simulink model "BLDC_180deg_hall_misalign"  (R2024a)
settings: Solver=ode15s  StartTime=0.0  StopTime=10  RelTol=1e-3
undefined symbols (not defined in the file or in its folder): HallError1, HallError2, HallError3, WrappedHallError1
libraries: simulink x10, dspswit3 x2, slpidlib x1
settings Model: Creator=matthewhasman  LastModifiedBy=matthewhasman

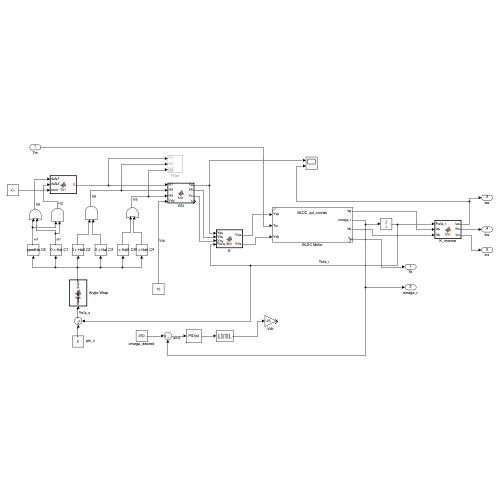
[thumbnail: Simulink's stored preview of the top-level diagram]
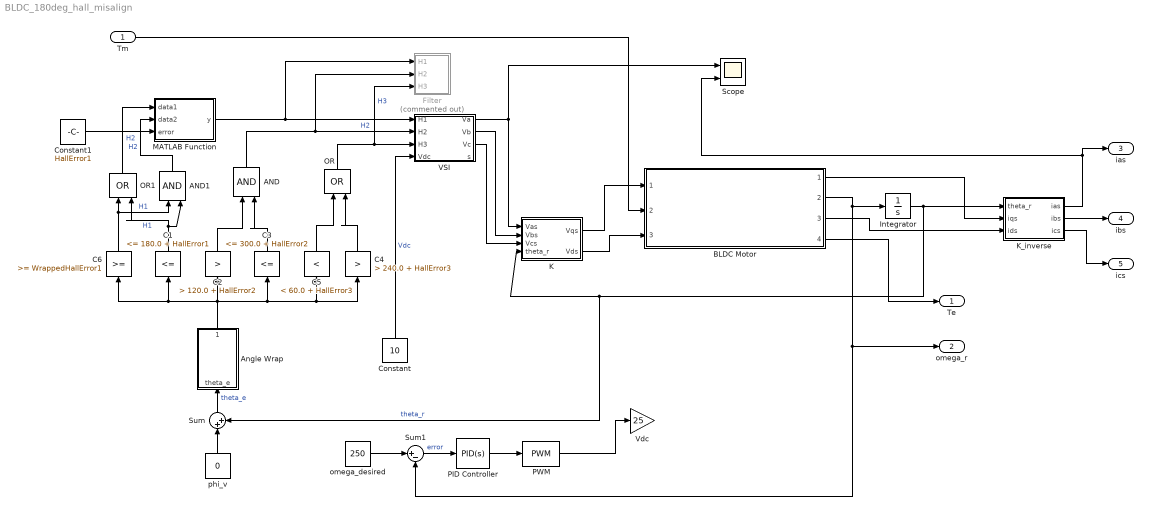
== system BLDC_180deg_hall_misalign ==
  Tm : Inport
  AND : Logic  IconShape=distinctive  AllPortsSameDT=off  OutDataTypeStr=boolean
  AND1 : Logic  IconShape=distinctive  AllPortsSameDT=off  OutDataTypeStr=boolean
  Angle Wrap : MATLAB Function  TreatAsAtomicUnit=on
  BLDC Motor : Subsystem  ReferencedSubsystem=BLDC_qd_coords
  C1 : simulink/Logic and Bit Operations/Compare To Constant  relop=<=  const=180.0 + HallError1  OutDataTypeStr=boolean
  C2 : simulink/Logic and Bit Operations/Compare To Constant  relop=>  const=120.0 + HallError2  OutDataTypeStr=boolean
  C3 : simulink/Logic and Bit Operations/Compare To Constant  relop=<=  const=300.0 + HallError2  OutDataTypeStr=boolean
  C4 : simulink/Logic and Bit Operations/Compare To Constant  relop=>  const=240.0 + HallError3  OutDataTypeStr=boolean
  C5 : simulink/Logic and Bit Operations/Compare To Constant  relop=<  const=60.0 + HallError3  OutDataTypeStr=boolean
  C6 : simulink/Logic and Bit Operations/Compare To Constant  relop=>=  const=WrappedHallError1  OutDataTypeStr=boolean
  Constant : Constant  Value=10
  Constant1 : Constant  Value=HallError1
  Filter : Subsystem  Commented=on
  Integrator : Integrator
  K : MATLAB Function  TreatAsAtomicUnit=on
  K_inverse : MATLAB Function  TreatAsAtomicUnit=on
  MATLAB Function : MATLAB Function  TreatAsAtomicUnit=on
  OR : Logic  Operator=OR  IconShape=distinctive  AllPortsSameDT=off  OutDataTypeStr=boolean
  OR1 : Logic  Operator=OR  IconShape=distinctive  AllPortsSameDT=off  OutDataTypeStr=boolean
  PID Controller : slpidlib/PID Controller  Controller=PID  Form=Parallel  TimeDomain=Continuous-time  UseExternalTs=off  SampleTime=-1  IntegratorMethod=Forward Euler  FilterMethod=Forward Euler  ControllerParametersSource=internal  P=8  I=5  UseKiTs=off  D=1  UseExternalDerivativeSource=off  N=100  UseFilter=on  TunerSelectOption=Transfer Function Based (PID Tuner App)  InitialConditionSource=internal  InitialConditionForIntegrator=0  InitialConditionForFilter=0  DifferentiatorICPrevScaledInput=0  ExternalReset=none  TrackingMode=off  Kt=1  LimitOutput=off  SatLimitsSource=internal  UpperSaturationLimit=inf  LowerSaturationLimit=-inf  LinearizeAsGain=on  AntiWindupMode=none  Kb=1  LimitIntegrator=off  UpperIntegratorSaturationLimit=inf  LowerIntegratorSaturationLimit=-inf  POutMin=[]  POutMax=[]  IOutMin=[]  IOutMax=[]  DOutMin=[]  DOutMax=[]  NOutMin=[]  NOutMax=[]  SumOutMin=[]  SumOutMax=[]  SaturationOutMin=[]  SaturationOutMax=[]  PParamMin=[]  PParamMax=[]  IParamMin=[]  IParamMax=[]  DParamMin=[]  DParamMax=[]  NParamMin=[]  NParamMax=[]  KbParamMin=[]  KbParamMax=[]  KtParamMin=[]  KtParamMax=[]  KbOutMin=[]  KbOutMax=[]  KtOutMin=[]  KtOutMax=[]  IntegratorOutMin=[]  IntegratorOutMax=[]  FilterOutMin=[]  FilterOutMax=[]  SumI1OutMin=[]  SumI1OutMax=[]  SumI2OutMin=[]  SumI2OutMax=[]  SumI3OutMin=[]  SumI3OutMax=[]  SumI4OutMin=[]  SumI4OutMax=[]  SumDOutMin=[]  SumDOutMax=[]  DifferentiatorOutMin=[]  DifferentiatorOutMax=[]  FilterDiffOutCoefMin=[]  FilterDiffOutCoefMax=[]  ReciprocalOutMin=[]  ReciprocalOutMax=[]  SumDenOutMin=[]  SumDenOutMax=[]  SumNumOutMin=[]  SumNumOutMax=[]  DivideOutMin=[]  DivideOutMax=[]  UdiffTsProdOutMin=[]  UdiffTsProdOutMax=[]  NTsProdOutMin=[]  NTsProdOutMax=[]  UintegralTsProdOutMin=[]  UintegralTsProdOutMax=[]  UngainTsProdOutMin=[]  UngainTsProdOutMax=[]  ClampingZeroOutDataTypeStr=Inherit: Inherit via back propagation  ClampingZeroOutMin=[]  ClampingZeroOutMax=[]  FilterDenConstantOutDataTypeStr=Inherit: Inherit via back propagation  FilterDenConstantOutMin=[]  FilterDenConstantOutMax=[]  PCopyOutDataTypeStr=Inherit: Inherit via back propagation  PCopyOutMin=[]  PCopyOutMax=[]  NCopyOutDataTypeStr=Inherit: Inherit via back propagation  NCopyOutMin=[]  NCopyOutMax=[]  IntegratorContinuousStateAttributes=''  IntegratorStateMustResolveToSignalObject=off  IntegratorRTWStateStorageClass=Auto  FilterContinuousStateAttributes=''  FilterStateMustResolveToSignalObject=off  FilterRTWStateStorageClass=Auto  ParallelPVariant=InternalParameters  IdealPVariant=Disabled  IVariant=InternalParameters  DVariant=InternalParameters  IntegratorVariant=Continuous  SatVariant=Disabled  AWVariant=Passthrough  PCopyVariant=Disabled  TRVariant=Disabled  FdbkBlocksVariant=Forward  IdealPFdbkVariant=Disabled  SatFdbkVariant=Disabled  DerivativeFilterVariant=ContFilter  NVariant=InternalParameters  NCopyVariant=Disabled  FilterICVariant=InternalICsFilter  IntegratorICVariant=InternalICs  ExternalResetVariant=Disabled  TRSumVariant=Passthrough  SumFdbkVariant=Disabled  SumVariant=Sum_PID  TsampFilterVariant=InternalTs  TsampNgainVariant=Passthrough  TsampIntegralVariant=Disabled_SignalSpec  ExternalSaturationOutDataTypeStr=Inherit: Same as second input  DerivativeSourceVariant=ErrorSignal
  PWM : simulink/Discontinuities/PWM  DisableCoverage=on  Period=0.0001  InitialDelay=0  DisallowZeroDutyCycle=off  RunAtFixedTimeIntervals=off  SampleTime=0.1
  Scope : Scope  NumInputPorts=2
  Sum : Sum  Inputs=|++
  Sum1 : Sum  Inputs=|+-
  VSI : MATLAB Function  TreatAsAtomicUnit=on
  Vdc : Gain  Gain=25
  omega_desired : Constant  Value=250
  phi_v : Constant  Value=0
  Te : Outport
  omega_r : Outport  Port=2
  ias : Outport  Port=3
  ibs : Outport  Port=4
  ics : Outport  Port=5
  wires:
  Integrator/1 -> K_inverse/1(theta_r), K/4(theta_r), Sum/2  "theta_r"
  BLDC Motor/1 -> K_inverse/2(iqs)
  BLDC Motor/3 -> K_inverse/3(ids)
  K/1(Vqs) -> BLDC Motor/1
  Tm/1 -> BLDC Motor/2
  phi_v/1 -> Sum/1
  VSI/1(Va) -> K/1(Vas), Scope/1
  VSI/2(Vb) -> K/2(Vbs)
  VSI/3(Vc) -> K/3(Vcs)
  omega_desired/1 -> Sum1/1
  Sum1/1 -> PID Controller/1  "error"
  PID Controller/1 -> PWM/1
  PWM/1 -> Vdc/1
  Constant/1 -> VSI/4(Vdc)  "Vdc"
  K/2(Vds) -> BLDC Motor/3
  Sum/1 -> Angle Wrap/1(theta_e)  "theta_e"
  Angle Wrap/1(wrapped_theta) -> C2/1, C5/1, C4/1, C3/1, C6/1, C1/1
  C2/1 -> AND/1
  C3/1 -> AND/2
  AND/1 -> Filter/2(H2), VSI/2(H2)  "H2"
  C5/1 -> OR/1
  C4/1 -> OR/2
  OR/1 -> Filter/3(H3), VSI/3(H3)  "H3"
  BLDC Motor/2 -> omega_r/1, Sum1/2, Integrator/1
  BLDC Motor/4 -> Te/1
  K_inverse/1(ias) -> Scope/2, ias/1
  K_inverse/2(ibs) -> ibs/1
  K_inverse/3(ics) -> ics/1
  C6/1 -> AND1/1, OR1/1  "H1"
  C1/1 -> AND1/2, OR1/2  "H1"
  MATLAB Function/1(y) -> Filter/1(H1), VSI/1(H1)
  OR1/1 -> MATLAB Function/1(data1)  "H2"
  AND1/1 -> MATLAB Function/2(data2)  "H2"
  Constant1/1 -> MATLAB Function/3(error)

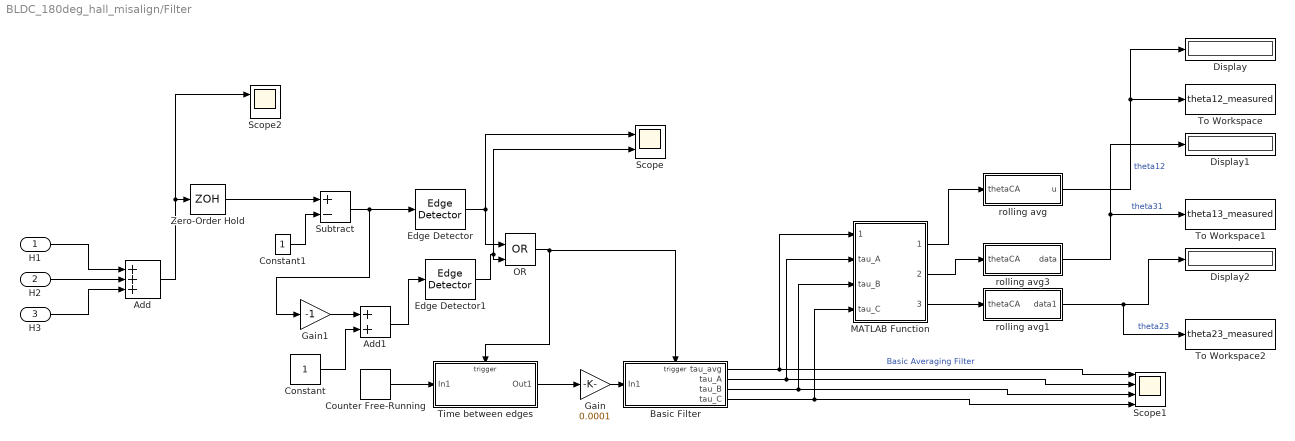
== system BLDC_180deg_hall_misalign/Filter ==
  H1 : Inport
  H2 : Inport  Port=2
  H3 : Inport  Port=3
  Add : Sum  Inputs=+++
  Add1 : Sum
  Basic Filter : Subsystem  TreatAsAtomicUnit=on
  Constant : Constant
  Constant1 : Constant
  Counter Free-Running : simulink/Sources/Counter Free-Running  NumBits=32  tsamp=0.0001
  Display : Display
  Display1 : Display
  Display2 : Display
  Edge Detector : dspswit3/Edge Detector  InputProcessing=Columns as channels (frame based)
  Edge Detector1 : dspswit3/Edge Detector  InputProcessing=Columns as channels (frame based)
  Gain : Gain  Gain=0.0001
  Gain1 : Gain  Gain=-1
  MATLAB Function : MATLAB Function  TreatAsAtomicUnit=on
  OR : Logic  Operator=OR  IconShape=distinctive  AllPortsSameDT=off  OutDataTypeStr=boolean
  Scope : Scope  NumInputPorts=2
  Scope1 : Scope  NumInputPorts=4
  Scope2 : Scope  NumInputPorts=2
  Subtract : Sum  Inputs=+-
  Time between edges : Subsystem  TreatAsAtomicUnit=on
  To Workspace : ToWorkspace  VariableName=theta12_measured  SaveFormat=Timeseries  SampleTime=-1
  To Workspace1 : ToWorkspace  VariableName=theta13_measured  SaveFormat=Timeseries  SampleTime=-1
  To Workspace2 : ToWorkspace  VariableName=theta23_measured  SaveFormat=Timeseries  SampleTime=-1
  Zero-Order Hold : ZeroOrderHold  SampleTime=0.00001
  rolling avg : Subsystem
  rolling avg1 : Subsystem
  rolling avg3 : Subsystem
  wires:
  H3/1 -> Add/3
  Counter Free-Running/1 -> Time between edges/1(In1)
  H1/1 -> Add/1
  Constant1/1 -> Subtract/2
  Add/1 -> Scope2/1, Zero-Order Hold/1
  Subtract/1 -> Gain1/1, Edge Detector/1
  H2/1 -> Add/2
  Zero-Order Hold/1 -> Subtract/1
  Basic Filter/1(tau_avg) -> MATLAB Function/1(tau_avg), Scope1/1  "Basic Averaging Filter"
  Edge Detector/1 -> OR/1, Scope/1
  Basic Filter/2(tau_A) -> MATLAB Function/2(tau_A), Scope1/2
  Basic Filter/3(tau_B) -> MATLAB Function/3(tau_B), Scope1/3
  Basic Filter/4(tau_C) -> MATLAB Function/4(tau_C), Scope1/4
  Time between edges/1(Out1) -> Gain/1
  Gain/1 -> Basic Filter/1(In1)
  Edge Detector1/1 -> Scope/2, OR/2
  OR/1 -> Basic Filter/Trigger, Time between edges/Trigger
  Gain1/1 -> Add1/1
  Add1/1 -> Edge Detector1/1
  Constant/1 -> Add1/2
  MATLAB Function/1(thetaCA) -> rolling avg/1(thetaCA)
  rolling avg/1(u) -> To Workspace/1, Display/1  "theta12"
  MATLAB Function/2(thetaBC) -> rolling avg3/1(thetaCA)
  rolling avg3/1(data) -> To Workspace1/1, Display1/1  "theta31"
  MATLAB Function/3(thetaAB) -> rolling avg1/1(thetaCA)
  rolling avg1/1(data1) -> Display2/1, To Workspace2/1  "theta23"

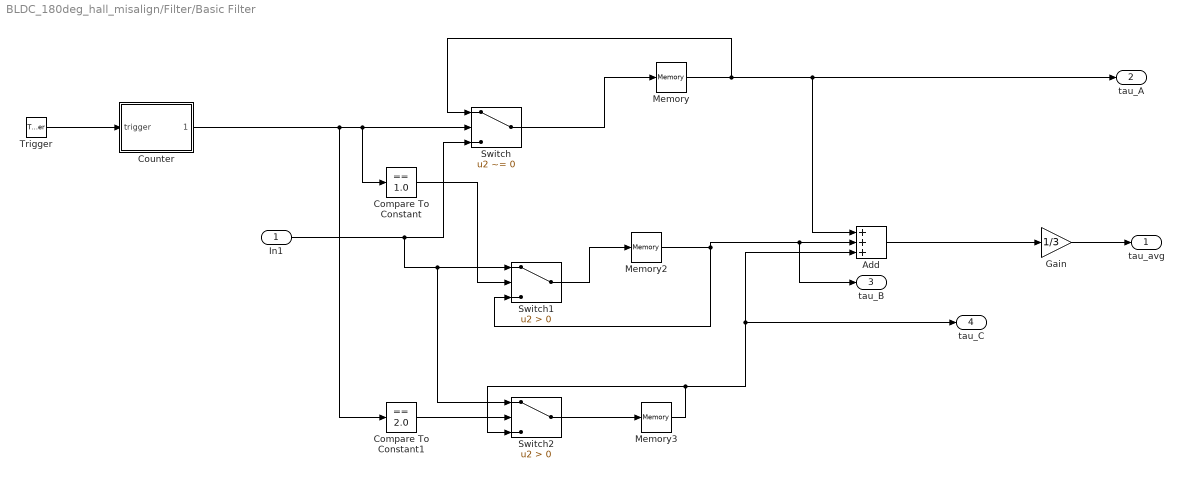
== system BLDC_180deg_hall_misalign/Filter/Basic Filter ==
  In1 : Inport
  Trigger : TriggerPort  VariantControl=(inherit)  ShowOutputPort=on
  Add : Sum  Inputs=+++
  Compare To Constant : simulink/Logic and Bit Operations/Compare To Constant  relop===  const=1.0  OutDataTypeStr=uint8
  Compare To Constant1 : simulink/Logic and Bit Operations/Compare To Constant  relop===  const=2.0  OutDataTypeStr=uint8
  Counter : MATLAB Function  TreatAsAtomicUnit=on
  Gain : Gain  Gain=1/3
  Memory : Memory  InheritSampleTime=on
  Memory2 : Memory  InheritSampleTime=on
  Memory3 : Memory  InheritSampleTime=on
  Switch : Switch  Criteria=u2 ~= 0  SaturateOnIntegerOverflow=off  InputSameDT=off
  Switch1 : Switch  Criteria=u2 > Threshold  SaturateOnIntegerOverflow=off  InputSameDT=off
  Switch2 : Switch  Criteria=u2 > Threshold  SaturateOnIntegerOverflow=off  InputSameDT=off
  tau_avg : Outport
  tau_A : Outport  Port=2
  tau_B : Outport  Port=3
  tau_C : Outport  Port=4
  wires:
  Add/1 -> Gain/1
  Gain/1 -> tau_avg/1
  Trigger/1 -> Counter/1(trigger)
  Counter/1(countOut) -> Compare To Constant1/1, Switch/2, Compare To Constant/1
  In1/1 -> Switch2/1, Switch1/1, Switch/3
  Switch/1 -> Memory/1
  Compare To Constant/1 -> Switch1/2
  Switch1/1 -> Memory2/1
  Memory2/1 -> tau_B/1, Add/2, Switch1/3
  Compare To Constant1/1 -> Switch2/2
  Switch2/1 -> Memory3/1
  Memory3/1 -> Switch2/3, tau_C/1, Add/3
  Memory/1 -> Switch/1, tau_A/1, Add/1

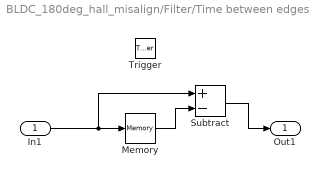
== system BLDC_180deg_hall_misalign/Filter/Time between edges ==
  In1 : Inport
  Trigger : TriggerPort  VariantControl=(inherit)
  Memory : Memory  InheritSampleTime=on
  Subtract : Sum  Inputs=+-
  Out1 : Outport
  wires:
  In1/1 -> Subtract/1, Memory/1
  Memory/1 -> Subtract/2
  Subtract/1 -> Out1/1

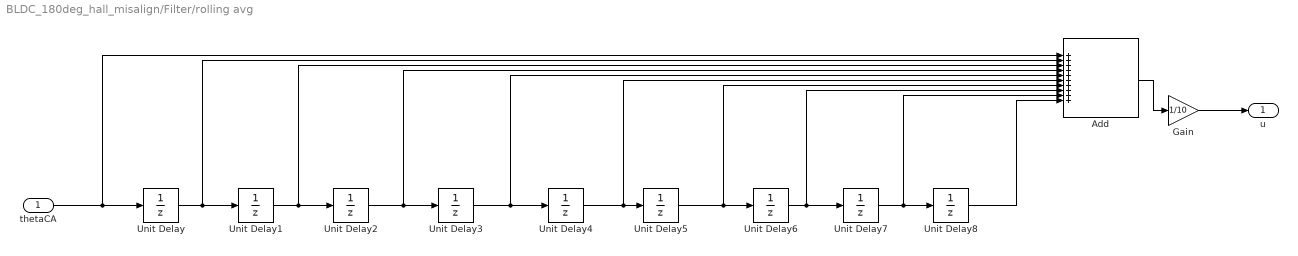
== system BLDC_180deg_hall_misalign/Filter/rolling avg ==
  thetaCA : Inport
  Add : Sum  Inputs=++++++++++
  Gain : Gain  Gain=1/10
  Unit Delay{,1..8} (9 alike) : UnitDelay  SampleTime=0.05  HasFrameUpgradeWarning=on
  u : Outport
  wires:
  Unit Delay/1 -> Unit Delay1/1, Add/2
  thetaCA/1 -> Unit Delay/1, Add/1
  Unit Delay2/1 -> Unit Delay3/1, Add/4
  Unit Delay3/1 -> Unit Delay4/1, Add/5
  Add/1 -> Gain/1
  Gain/1 -> u/1
  Unit Delay1/1 -> Unit Delay2/1, Add/3
  Unit Delay4/1 -> Unit Delay5/1, Add/6
  Unit Delay5/1 -> Add/7, Unit Delay6/1
  Unit Delay6/1 -> Add/8, Unit Delay7/1
  Unit Delay7/1 -> Add/9, Unit Delay8/1
  Unit Delay8/1 -> Add/10

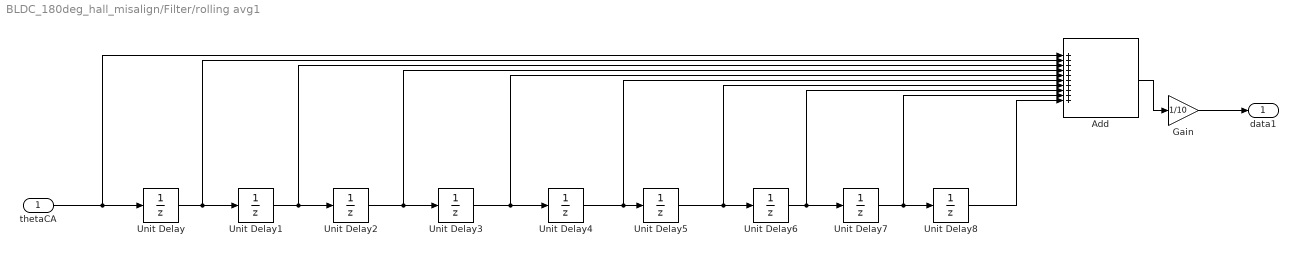
== system BLDC_180deg_hall_misalign/Filter/rolling avg1 ==
  thetaCA : Inport
  Add : Sum  Inputs=++++++++++
  Gain : Gain  Gain=1/10
  Unit Delay{,1..8} (9 alike) : UnitDelay  SampleTime=0.05  HasFrameUpgradeWarning=on
  data1 : Outport
  wires:
  Unit Delay/1 -> Unit Delay1/1, Add/2
  thetaCA/1 -> Unit Delay/1, Add/1
  Unit Delay2/1 -> Unit Delay3/1, Add/4
  Unit Delay3/1 -> Unit Delay4/1, Add/5
  Add/1 -> Gain/1
  Gain/1 -> data1/1
  Unit Delay1/1 -> Unit Delay2/1, Add/3
  Unit Delay4/1 -> Unit Delay5/1, Add/6
  Unit Delay5/1 -> Add/7, Unit Delay6/1
  Unit Delay6/1 -> Add/8, Unit Delay7/1
  Unit Delay7/1 -> Add/9, Unit Delay8/1
  Unit Delay8/1 -> Add/10

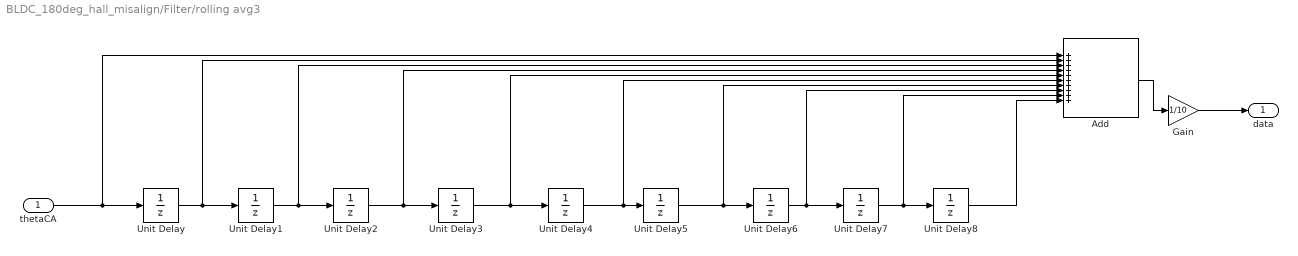
== system BLDC_180deg_hall_misalign/Filter/rolling avg3 ==
  thetaCA : Inport
  Add : Sum  Inputs=++++++++++
  Gain : Gain  Gain=1/10
  Unit Delay{,1..8} (9 alike) : UnitDelay  SampleTime=0.05  HasFrameUpgradeWarning=on
  data : Outport
  wires:
  Unit Delay/1 -> Unit Delay1/1, Add/2
  thetaCA/1 -> Unit Delay/1, Add/1
  Unit Delay2/1 -> Unit Delay3/1, Add/4
  Unit Delay3/1 -> Unit Delay4/1, Add/5
  Add/1 -> Gain/1
  Gain/1 -> data/1
  Unit Delay1/1 -> Unit Delay2/1, Add/3
  Unit Delay4/1 -> Unit Delay5/1, Add/6
  Unit Delay5/1 -> Add/7, Unit Delay6/1
  Unit Delay6/1 -> Add/8, Unit Delay7/1
  Unit Delay7/1 -> Add/9, Unit Delay8/1
  Unit Delay8/1 -> Add/10

== matlab function BLDC_180deg_hall_misalign/K ==
  data: Vas input; Vqs output; Vbs input; Vcs input; Vds output; theta_r input
function [Vqs, Vds] = fcn(Vas, Vbs, Vcs, theta_r)
offset = 2*pi/3;
k = (2/3)*[cos(theta_r), cos(theta_r - offset), cos(theta_r + offset);
           sin(theta_r), sin(theta_r - offset), sin(theta_r + offset)];

qds_voltage = k * [Vas; Vbs; Vcs];

Vqs = qds_voltage(1);
Vds = qds_voltage(2);

end

== matlab function BLDC_180deg_hall_misalign/K_inverse ==
  data: theta_r input; ias output; iqs input; ids input; ibs output; ics output
function [ias, ibs, ics] = fcn(theta_r, iqs, ids)
offset = 2*pi/3;
k_inverse = [cos(theta_r), sin(theta_r);
             cos(theta_r - offset), sin(theta_r - offset);
             cos(theta_r + offset), sin(theta_r + offset)];

abc_currents = k_inverse * [iqs; ids];

ias = abc_currents(1);
ibs = abc_currents(2);
ics = abc_currents(3);

end

== matlab function BLDC_180deg_hall_misalign/Angle Wrap ==
  data: theta_e input; wrapped_theta output
function wrapped_theta = fcn(theta_e)

wrapped_theta = wrapTo2Pi(theta_e) * 180 / pi;

== matlab function BLDC_180deg_hall_misalign/VSI ==
  data: Va output; H1 input; H2 input; H3 input; Vb output; Vc output; Vdc input; s output
function [Va, Vb, Vc, s] = fcn(H1, H2, H3, Vdc)

% Initialize T1, T2, T3
T1 = 0;
T2 = 0;
T3 = 0;
s=0;

% Determine T1, T2, T3 based on theta_e
if (H1 && H3)
    [T1, T2, T3] = deal(1, 0, 0);
    s=0;
elseif (H1 && ~H2 && ~H3)
    [T1, T2, T3] = deal(1, 1, 0);
    s=1;
elseif (H2 && H1)
    [T1, T2, T3] = deal(0, 1, 0);
    s=2;
elseif (H2 && ~H1 && ~H3)
    [T1, T2, T3] = deal(0, 1, 1);
    s=3;
elseif (H2 && H3)
    [T1, T2, T3] = deal(0, 0, 1);
    s=4;
else
    [T1, T2, T3] = deal(1, 0, 1);
    s=5;
end

% % Determine T1, T2, T3 based on theta_e
% if (H1 && H3)
%     [T1, T2, T3] = deal(1, 0, 1);
%     s=0;
% elseif (H1)
%     [T1, T2, T3] = deal(1, 0, 0);
%     s=1;
% elseif (H2 && H1)
%     [T1, T2, T3] = deal(1, 1, 0);
%     s=2;
% elseif (H2)
%     [T1, T2, T3] = deal(0, 1, 0);
%     s=3;
% elseif (H2 && H3)
%     [T1, T2, T3] = deal(0, 1, 1);
%     s=4;
% else
%     [T1, T2, T3] = deal(0, 0, 1);
%     s=5;
% end

% Matrix A for transformations
A = [2/3, -1/3, -1/3;
     -1/3, 2/3, -1/3;
     -1/3, -1/3, 2/3;];

% Create T vector
T = [T1; T2; T3];

% Compute Vabc
Vabc = Vdc * A * T;

Va = Vabc(1);
Vb = Vabc(2); 
Vc = Vabc(3); 

end

== matlab function BLDC_180deg_hall_misalign/MATLAB Function ==
  data: data1 input; y output; data2 input; error input
function y = fcn(data1, data2, error)

if error > 0
    y = data2;

else 
    y = data1;

end

== matlab function BLDC_180deg_hall_misalign/Filter/Basic Filter/Counter ==
  data: trigger input; countOut output
function countOut = simpleCounter(trigger)
    persistent counter;  % Persistent variable to hold the count
    if isempty(counter)   % Initialize on the first call
        counter = 0;
    end
    
    if trigger           % Increment on trigger
        counter = mod(counter + 1, 3);  % Wraps around after 2
    end
    
    countOut = counter;  % Output the current count
end

== matlab function BLDC_180deg_hall_misalign/Filter/MATLAB Function ==
  data: tau_avg input; thetaCA output; tau_A input; tau_B input; tau_C input; thetaBC output; thetaAB output
function [thetaCA, thetaBC, thetaAB] = fcn(tau_avg, tau_A, tau_B, tau_C)
    % Ensure inputs are treated as double
    tau_avg = double(tau_avg);
    tau_A = double(tau_A);
    tau_B = double(tau_B);
    tau_C = double(tau_C);
    
    % Initialize outputs to avoid unassigned output error
    thetaCA = 0;
    thetaBC = 0;
    thetaAB = 0;

    % Calculate theta values based on the input parameters
    thetaCA = 60*(tau_A - tau_avg)/(tau_avg);
    thetaBC = 60*(tau_B - tau_avg)/(tau_avg);
    thetaAB = 60*(tau_C - tau_avg)/(tau_avg);
end
